simulink model "lab1v1Orozco"  (R2017b)
settings: Solver=VariableStepAuto  StartTime=0.0  StopTime=0.002  RelTol=1e-3
libraries: commrandsrc3 x4
settings Model: Creator=n0b0dy  LastModifiedBy=user

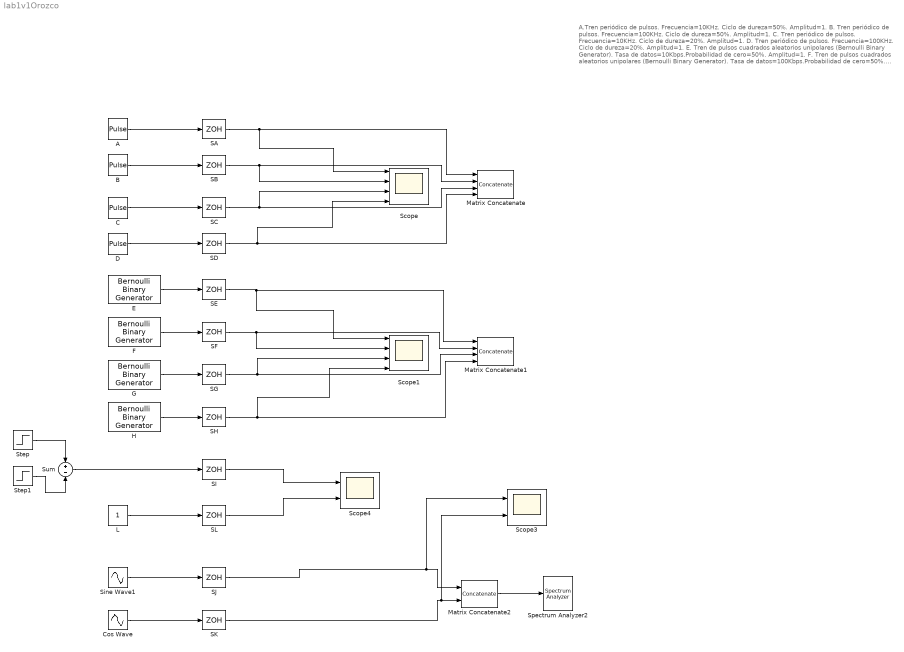
== system lab1v1Orozco ==
  note: A.Tren periódico de pulsos. Frecuencia=10KHz. Ciclo de dureza=50%. Amplitud=1.
      | B. Tren periódico de pulsos. Frecuencia=100KHz. Ciclo de dureza=50%. Amplitud=1.
      | C. Tren periódico de pulsos. Frecuencia=10KHz. Ciclo de dureza=20%. Amplitud=1.
      | D. Tren periódico de pulsos. Frecuencia=100KHz. Ciclo de dureza=20%. Amplitud=1.
      | E. Tren de pulsos cuadrados aleatorios unipolares (Bernoulli Binary Generator). Tasa de datos=10Kbps.Probabilidad de cero=50%. Amplitud=1.
      | F. Tren de pulsos cuadrados aleatorios unipolares (Bernoulli Binary Generator). Tasa de datos=100Kbps.Probabilidad de cero=50%. Amplitud=1.
      | G. Tren de pulsos cuadrados aleatorios unipolares (Bernoulli Binary Generator). Tasa de datos=10Kbps.Probabilidad de cero=30%. Amplitud=1.
      | H. Tren de pulsos cuadrados aleatorios unipolares (Bernoulli Binary Generator). Tasa de datos=100Kbps.Probabilidad de cero=30%. Amplitud=1.
      | I. Un pulso rectangular de amplitud 3, iniciando en t0=0.5s y terminando en t1=0.7s
      | J. Seno. Frecuencia=1Khz. Amplitud=1.
      | K. Coseno. Frecuencia=1Khz. Amplitud=1.
      | L. Señal constante. Amplitud=1
  A : DiscretePulseGenerator  PulseType=Time based  Period=1/10E3  PulseWidth=50
  B : DiscretePulseGenerator  PulseType=Time based  Period=1/100E3  PulseWidth=50  VectorParams1D=off
  C : DiscretePulseGenerator  PulseType=Time based  Period=1/10E3  PulseWidth=20
  Cos Wave : Sin  Frequency=1e3*2*pi  Phase=pi/2  SampleTime=0
      settings: AttributesFormatString=|
      | Frecuency = %<Frequency>
      | Phase = %<Phase>
  D : DiscretePulseGenerator  PulseType=Time based  Period=1/100E3  PulseWidth=20
  E : commrandsrc3/Bernoulli Binary Generator  ProbabilityOfZero=0.5  SeedSource=Parameter  Seed=1  SampleTime=1/10e3  SamplesPerFrame=1  OutputDataType=double  SimulateUsing=Interpreted execution
  F : commrandsrc3/Bernoulli Binary Generator  ProbabilityOfZero=0.5  SeedSource=Parameter  Seed=1  SampleTime=1/100e3  SamplesPerFrame=1  OutputDataType=double  SimulateUsing=Interpreted execution
  G : commrandsrc3/Bernoulli Binary Generator  ProbabilityOfZero=0.3  SeedSource=Parameter  Seed=1  SampleTime=1/10e3  SamplesPerFrame=1  OutputDataType=double  SimulateUsing=Interpreted execution
  H : commrandsrc3/Bernoulli Binary Generator  ProbabilityOfZero=0.3  SeedSource=Parameter  Seed=1  SampleTime=1/100e3  SamplesPerFrame=1  OutputDataType=double  SimulateUsing=Interpreted execution
  L : Constant  SampleTime=1/(6*(1000*2*pi))
  Matrix Concatenate : Concatenate  NumInputs=4  Mode=Multidimensional array  ConcatenateDimension=2
  Matrix Concatenate1 : Concatenate  NumInputs=4  Mode=Multidimensional array  ConcatenateDimension=2
  Matrix Concatenate2 : Concatenate  Mode=Multidimensional array  ConcatenateDimension=2
  SA : ZeroOrderHold  SampleTime=1/(10*100e3)
  SB : ZeroOrderHold  SampleTime=1/(100*100e3)
  SC : ZeroOrderHold  SampleTime=1/(10*100e3)
  SD : ZeroOrderHold  SampleTime=1/(100*100e3)
  SE : ZeroOrderHold  SampleTime=1/(10*100e3)
  SF : ZeroOrderHold  SampleTime=1/(100*100e3)
  SG : ZeroOrderHold  SampleTime=1/(10*100e3)
  SH : ZeroOrderHold  SampleTime=1/(100*100e3)
  SI : ZeroOrderHold  SampleTime=1/10e3
  SJ : ZeroOrderHold  SampleTime=1/(1*100e3)
  SK : ZeroOrderHold  SampleTime=1/100e3
  SL : ZeroOrderHold  SampleTime=1/6e3
  Scope : Scope  NumInputPorts=4
  Scope1 : Scope  NumInputPorts=4
  Scope3 : Scope  NumInputPorts=2
  Scope4 : Scope  NumInputPorts=2
  Sine Wave1 : Sin  Frequency=1e3*2*pi  SampleTime=0
      settings: AttributesFormatString=|
      | Frecuency = %<Frequency>
      | Phase = %<Phase>
  Spectrum Analyzer2 : SpectrumAnalyzer
  Step : Step  Time=0.5  After=3  SampleTime=1e-3
      settings: AttributesFormatString=Step Time = %<Time>
  Step1 : Step  Time=0.7  After=3  SampleTime=1e-3
      settings: AttributesFormatString=Step Time = %<Time>
  Sum : Sum  Inputs=+|-
  wires:
  A/1 -> SA/1
  E/1 -> SE/1
  F/1 -> SF/1
  G/1 -> SG/1
  H/1 -> SH/1
  B/1 -> SB/1
  C/1 -> SC/1
  D/1 -> SD/1
  SA/1 -> Scope/1, Matrix Concatenate/1
  SD/1 -> Matrix Concatenate/4, Scope/4
  SH/1 -> Matrix Concatenate1/4, Scope1/4
  SG/1 -> Matrix Concatenate1/3, Scope1/3
  SF/1 -> Matrix Concatenate1/2, Scope1/2
  SE/1 -> Matrix Concatenate1/1, Scope1/1
  SC/1 -> Scope/3, Matrix Concatenate/3
  SB/1 -> Scope/2, Matrix Concatenate/2
  L/1 -> SL/1
  Sine Wave1/1 -> SJ/1
  Cos Wave/1 -> SK/1
  Step1/1 -> Sum/2
  Step/1 -> Sum/1
  Sum/1 -> SI/1
  SI/1 -> Scope4/1
  SL/1 -> Scope4/2
  Matrix Concatenate2/1 -> Spectrum Analyzer2/1
  SJ/1 -> Scope3/1, Matrix Concatenate2/1
  SK/1 -> Scope3/2, Matrix Concatenate2/2
